simulink model "capacitor2"  (R2020a)
settings: Solver=VariableStepAuto  StartTime=0.0  StopTime=10.0  RelTol=1e-3
libraries: powerlib x8
settings Model: Creator=matt  LastModifiedBy=matt

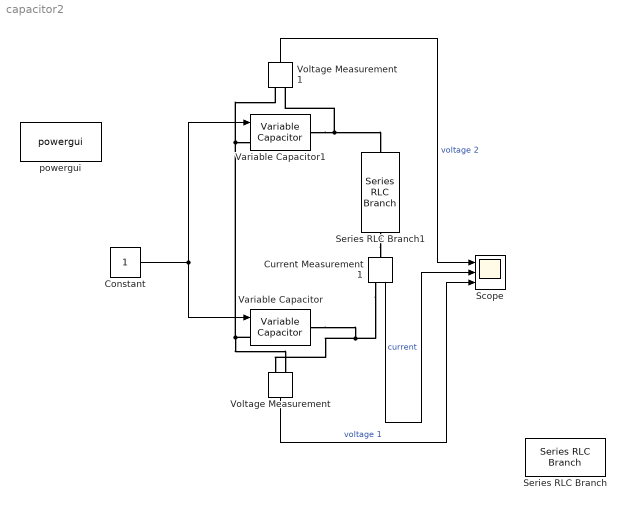
== system capacitor2 ==
  Constant : Constant
  Current Measurement1 : powerlib/Measurements/Current Measurement  PhasorSimulation=off  OutputType=Complex  PSBequivalent=0
  Scope : Scope  NumInputPorts=3
  Series RLC Branch : powerlib/Elements/Series RLC Branch  LConnTagsString=__new0  RConnTagsString=__new0  BranchType=RLC  Resistance=1  Inductance=1e-3  SetiL0=off  InitialCurrent=0  Capacitance=1e-6  Setx0=off  InitialVoltage=0  Measurements=None
  Series RLC Branch1 : powerlib/Elements/Series RLC Branch  LConnTagsString=__new0  RConnTagsString=__new0  BranchType=R  Resistance=1  Inductance=1e-3  SetiL0=off  InitialCurrent=0  Capacitance=1e-6  Setx0=off  InitialVoltage=0  Measurements=None
  Variable Capacitor : powerlib/Elements/Variable Capacitor  methode=Backward Euler  Cabsmin=1e-9  Initialize=on  vC0=12  C0=1  iC0=-12
      settings: SourceProductBaseCode=PS
  Variable Capacitor1 : powerlib/Elements/Variable Capacitor  methode=Backward Euler  Cabsmin=1e-9  Initialize=on  vC0=0  C0=1  iC0=12
      settings: SourceProductBaseCode=PS
  Voltage Measurement : powerlib/Measurements/Voltage Measurement  PhasorSimulation=off  OutputType=Complex  PSBequivalent=0
  Voltage Measurement1 : powerlib/Measurements/Voltage Measurement  PhasorSimulation=off  OutputType=Complex  PSBequivalent=0
  powergui : powerlib/powergui  Priority=1  SimulationMode=Discrete  SampleTime=50e-6  frequency=60  Iterations=50  frequencyindice=0  Pbase=100e6  ErrMax=1e-4  UnitsV=kV  UnitsW=MW  buscounter=0  FunctionMessages=off  echomessages=off  EnableUseOfTLC=off  CurrentSourceSwitches=off  DisableSnubberDevices=off  DisableRonSwitches=off  DisableVfSwitches=off  DisplayEquations=off  AutomaticDiscreteSolvers=off  SolverType=Tustin/Backward Euler (TBE)  Interpol=off  ExternalGateDelay=off  methode=off  Ts=100  x0status=blocks  SPID=on  SwTol=0  HookPort=off  NonlinearTolerance=1e-4  nMaxIteration=100  ContinueOnMaxIteration=off  RestoreLinks=warning  ResistiveCurrentMeasurement=off  Frange=[0:2:500]  Ylog=off  Xlog=on  ShowGrid=off  save=off  variable=ZData  structure=0  ZoomFFT=off  StartTime=0.0  cycles=1  DisplayStyle=1  fundamental=60  FreqAxis=off  MaxFrequency=1000  frequencyindicesteady=1  RmsSteady=1  display=off
  wires:
  Voltage Measurement/1 -> Scope/3  "voltage 1"
  Current Measurement1/1 -> Scope/2  "current"
  Constant/1 -> Variable Capacitor1/1, Variable Capacitor/1
  Voltage Measurement1/1 -> Scope/1  "voltage 2"
  connections:
  Current Measurement1/RConn1 -- Voltage Measurement/LConn2 -- Variable Capacitor/RConn1
  Variable Capacitor/LConn1 -- Voltage Measurement/LConn1 -- Voltage Measurement1/LConn1 -- Variable Capacitor1/LConn1
  Variable Capacitor1/RConn1 -- Voltage Measurement1/LConn2 -- Series RLC Branch1/LConn1
  Series RLC Branch1/RConn1 -- Current Measurement1/LConn1
